simulink library "HEV_lib"  (Simulink 7.7)
settings: Solver=ode45  SolverMode=SingleTasking  StartTime=0.0  StopTime=10.0  RelTol=1e-3
undefined symbols (not defined in the file): DiscIntNeverNeededParam, Hydride, magnitude, Metal, Nickel, Ts
libraries: powerlib x72, driveline x12, simulink_extras x8, electricdrivelib x7, simulink x6, powerlib_extras x2, HEV_lib x1
(part 1 of 3)
Description:
  | Copyright 2008-2011 The MathWorks, Inc.
settings Model: Creator=MathWorks  LastModifiedBy=xd1824

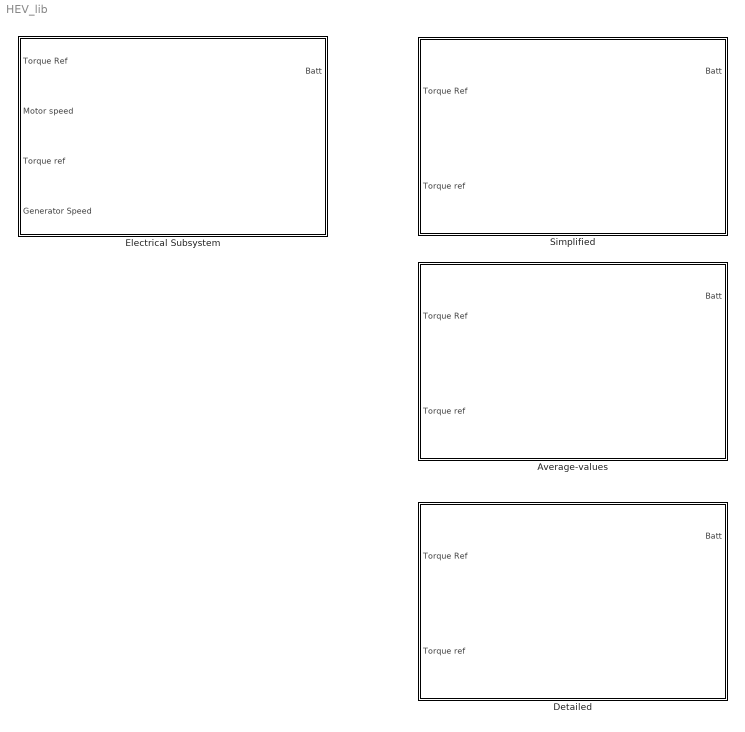
== system HEV_lib ==
  Average-values : Subsystem
      mask Display: image(imread('power_HEV_powertrain_electrical2.png'))
  Detailed : Subsystem
      mask Display: image(imread('power_HEV_powertrain_electrical2.png'))
  Electrical Subsystem : Subsystem  BlockChoice=Simplified
      settings: TemplateBlock=self  MemberBlocks=Average-values,Detailed,Simplified
      mask Display: image(imread('power_HEV_powertrain_electrical2.png'))
  Simplified : Subsystem
      mask Display: image(imread('power_HEV_powertrain_electrical2.png'))

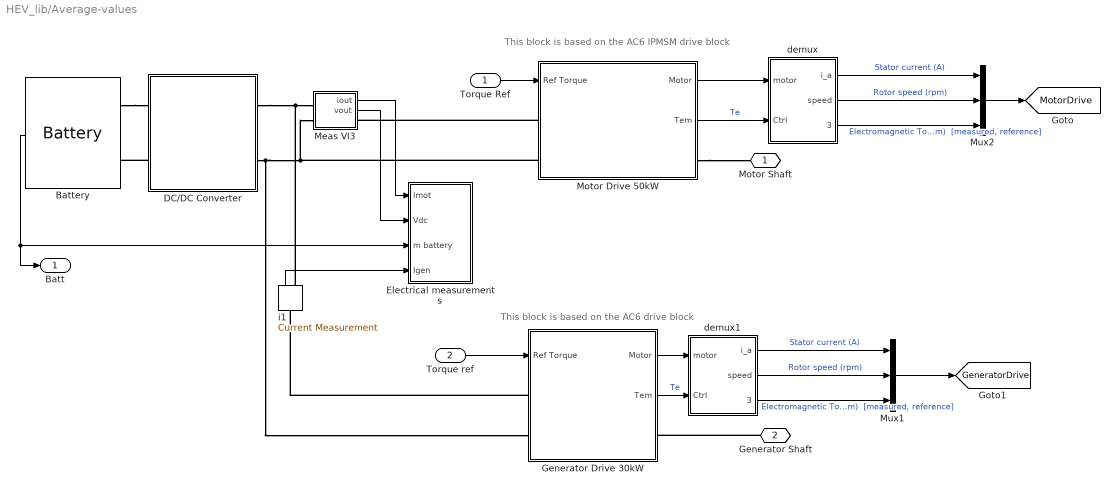
== system HEV_lib/Average-values ==
  note: This block is based on the
      | AC6 IPMSM drive block
  note: This block is based on the AC6
      | drive block
  Torque Ref : Inport
  Torque ref : Inport  Port=2
  Battery : electricdrivelib/Extra Sources/Battery  SystemSampleTime=-1  BatType=Nickel-Metal-Hydride  ShowDetailedParameters=off  NomV=200  NomQ=6.5  SOC=100  PresetModel=on  MaxQ=7  FullV=235.5932  Dis_rate=1.3  R=0.30769  Normal_OP=6.25  expZone="[216.9492           1.3]"  Dis_Char=off  current=[50 100]  Units=Time  Batt_Tr=30
  DC/DC Converter : Subsystem
      mask init:
      | [X1,X1m,X2,X2m,X3,X4,Y1,Y1m,Y2,Y2m,Y3,Y4,color1,color2]=spsdrivelogo;
      mask Display:
      | patch([X1 X1m],[Y1 Y1m],color1);
      | patch(X3,Y3,color2);
      | plot([X1 X1m X2 X2m X3 X4],[Y1 Y1m Y2 Y2m Y3 Y4]);
  Electrical measurements : Subsystem
  Generator Drive 30kW : Subsystem
      mask Display: image(imread('power_HEV_powertrain_syncgenerator.jpg'))
  Meas VI3 : Subsystem
  Motor Drive 50kW : Subsystem
      mask Display: image(imread('power_HEV_powertrain_syncmotor.jpg'))
  Mux1 : Mux  Inputs=3
  Mux2 : Mux  Inputs=3
  demux : Subsystem
  demux1 : Subsystem
  i1 : powerlib/Measurements/Current Measurement  SystemSampleTime=-1  PhasorSimulation=off  OutputType=Complex  PSBequivalent=0
  Motor Shaft : PMIOPort  Port=1  Side=Right
  Generator Shaft : PMIOPort  Port=2  Side=Right
  Batt : Outport
  tag scope: GeneratorDrive=global, MotorDrive=global
  wires:
  i1/1 -> Electrical measurements/4(Igen)
  Meas VI3/2(vout) -> Electrical measurements/2(Vdc)
  Meas VI3/1(iout) -> Electrical measurements/1(Imot)
  Torque ref/1 -> Generator Drive 30kW/1(Ref Torque)
  Battery/1 -> Electrical measurements/3(m battery), Batt/1
  demux1/2(speed) -> Mux1/2  "Rotor speed (rpm)"
  demux1/3(Torque) -> Mux1/3  "Electromagnetic Torque (Nm)  [measured, reference]"
  demux1/1(i_a) -> Mux1/1  "Stator current (A)"
  Generator Drive 30kW/1(Motor) -> demux1/1(motor)
  Torque Ref/1 -> Motor Drive 50kW/1(Ref Torque)
  Motor Drive 50kW/1(Motor) -> demux/1(motor)
  demux/2(speed) -> Mux2/2  "Rotor speed (rpm)"
  demux/3(Torque) -> Mux2/3  "Electromagnetic Torque (Nm)  [measured, reference]"
  demux/1(i_a) -> Mux2/1  "Stator current (A)"
  Mux2/1 -> [MotorDrive]
  Mux1/1 -> [GeneratorDrive]
  Motor Drive 50kW/2(Tem) -> demux/2(Ctrl)  "Te"
  Generator Drive 30kW/2(Tem) -> demux1/2(Ctrl)  "Te"
  connections:
  DC/DC Converter/LConn2 -- Battery/LConn2
  Battery/LConn1 -- DC/DC Converter/LConn1
  Generator Shaft/RConn1 -- Generator Drive 30kW/RConn1
  Motor Drive 50kW/LConn1 -- Meas VI3/RConn1
  DC/DC Converter/RConn1 -- Meas VI3/LConn1 -- i1/RConn1
  Generator Drive 30kW/LConn1 -- i1/LConn1
  DC/DC Converter/RConn2 -- Generator Drive 30kW/LConn2 -- Motor Drive 50kW/LConn2 -- Meas VI3/LConn2
  Motor Drive 50kW/RConn1 -- Motor Shaft/RConn1

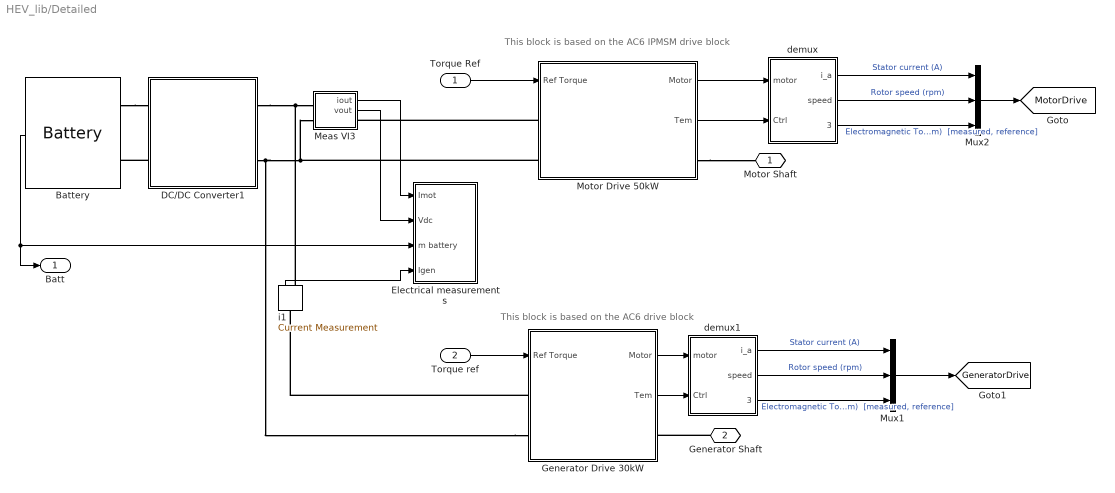
== system HEV_lib/Detailed ==
  note: This block is based on the AC6
      | drive block
  note: This block is based on the
      | AC6 IPMSM drive block
  Torque Ref : Inport
  Torque ref : Inport  Port=2
  Battery : electricdrivelib/Extra Sources/Battery  SystemSampleTime=-1  BatType=Nickel-Metal-Hydride  ShowDetailedParameters=off  NomV=200  NomQ=6.5  SOC=100  PresetModel=on  MaxQ=7  FullV=235.5932  Dis_rate=1.3  R=0.30769  Normal_OP=6.25  expZone="[216.9492           1.3]"  Dis_Char=off  current=[50 100]  Units=Time  Batt_Tr=30
  DC/DC Converter1 : Subsystem
      mask init:
      | [X1,X1m,X2,X2m,X3,X4,Y1,Y1m,Y2,Y2m,Y3,Y4,color1,color2]=spsdrivelogo;
      mask Display:
      | patch([X1 X1m],[Y1 Y1m],color1);
      | patch(X3,Y3,color2);
      | plot([X1 X1m X2 X2m X3 X4],[Y1 Y1m Y2 Y2m Y3 Y4]);
  Electrical measurements : Subsystem
  Generator Drive 30kW : Subsystem
      mask Display: image(imread('power_HEV_powertrain_syncgenerator.jpg'))
  Meas VI3 : Subsystem
  Motor Drive 50kW : Subsystem
      mask Display: image(imread('power_HEV_powertrain_syncmotor.jpg'))
  Mux1 : Mux  Inputs=3
  Mux2 : Mux  Inputs=3
  demux : Subsystem
  demux1 : Subsystem
  i1 : powerlib/Measurements/Current Measurement  SystemSampleTime=-1  PhasorSimulation=off  OutputType=Complex  PSBequivalent=0
  Motor Shaft : PMIOPort  Port=1  Side=Right
  Generator Shaft : PMIOPort  Port=2  Side=Right
  Batt : Outport
  tag scope: GeneratorDrive=global, MotorDrive=global
  wires:
  demux/1(i_a) -> Mux2/1  "Stator current (A)"
  demux/3(Torque) -> Mux2/3  "Electromagnetic Torque (Nm)  [measured, reference]"
  demux/2(speed) -> Mux2/2  "Rotor speed (rpm)"
  Motor Drive 50kW/2(Tem) -> demux/2(Ctrl)
  Motor Drive 50kW/1(Motor) -> demux/1(motor)
  Torque Ref/1 -> Motor Drive 50kW/1(Ref Torque)
  Generator Drive 30kW/2(Tem) -> demux1/2(Ctrl)
  Generator Drive 30kW/1(Motor) -> demux1/1(motor)
  demux1/1(i_a) -> Mux1/1  "Stator current (A)"
  demux1/3(Torque) -> Mux1/3  "Electromagnetic Torque (Nm)  [measured, reference]"
  demux1/2(speed) -> Mux1/2  "Rotor speed (rpm)"
  Battery/1 -> Batt/1, Electrical measurements/3(m battery)
  Torque ref/1 -> Generator Drive 30kW/1(Ref Torque)
  Meas VI3/1(iout) -> Electrical measurements/1(Imot)
  Meas VI3/2(vout) -> Electrical measurements/2(Vdc)
  i1/1 -> Electrical measurements/4(Igen)
  Mux2/1 -> [MotorDrive]
  Mux1/1 -> [GeneratorDrive]
  connections:
  Motor Drive 50kW/RConn1 -- Motor Shaft/RConn1
  Generator Drive 30kW/LConn2 -- Meas VI3/LConn2 -- Motor Drive 50kW/LConn2 -- DC/DC Converter1/RConn2
  Generator Drive 30kW/LConn1 -- i1/LConn1
  DC/DC Converter1/RConn1 -- i1/RConn1 -- Meas VI3/LConn1
  Motor Drive 50kW/LConn1 -- Meas VI3/RConn1
  Generator Shaft/RConn1 -- Generator Drive 30kW/RConn1
  Battery/LConn1 -- DC/DC Converter1/LConn1
  DC/DC Converter1/LConn2 -- Battery/LConn2

== system HEV_lib/Electrical Subsystem ==
  Torque Ref : Inport
  Motor speed : Inport  Port=2
  Torque ref : Inport  Port=3
  Generator Speed : Inport  Port=4
  Simplified : HEV_lib/Simplified  SystemSampleTime=-1
  Motor Shaft : PMIOPort  Port=1  Side=Right
  Generator Shaft : PMIOPort  Port=2  Side=Right
  Batt : Outport
  wires:
  Torque Ref/1 -> Simplified/1
  Motor speed/1 -> Simplified/2
  Torque ref/1 -> ?
  Generator Speed/1 -> ?
  Simplified/1 -> Batt/1
  connections:
  Simplified/RConn1 -- Motor Shaft/RConn1
  Simplified/RConn2 -- Generator Shaft/RConn1

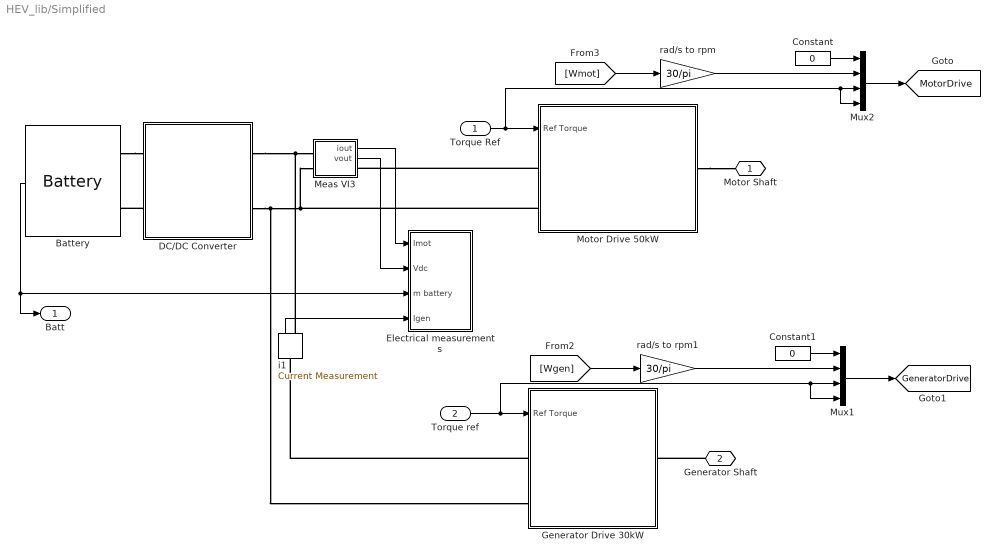
== system HEV_lib/Simplified ==
  Torque Ref : Inport
  Torque ref : Inport  Port=2
  Battery : electricdrivelib/Extra Sources/Battery  SystemSampleTime=-1  BatType=Nickel-Metal-Hydride  ShowDetailedParameters=off  NomV=200  NomQ=6.5  SOC=100  PresetModel=on  MaxQ=7  FullV=235.5932  Dis_rate=1.3  R=0.30769  Normal_OP=6.25  expZone="[216.9492           1.3]"  Dis_Char=off  current=[50 100]  Units=Time  Batt_Tr=30
  Constant : Constant  Value=0
  Constant1 : Constant  Value=0
  DC/DC Converter : Subsystem
      mask init:
      | [X1,X1m,X2,X2m,X3,X4,Y1,Y1m,Y2,Y2m,Y3,Y4,color1,color2]=spsdrivelogo;
      mask Display:
      | patch([X1 X1m],[Y1 Y1m],color1);
      | patch(X3,Y3,color2);
      | plot([X1 X1m X2 X2m X3 X4],[Y1 Y1m Y2 Y2m Y3 Y4]);
  Electrical measurements : Subsystem
  Generator Drive 30kW : Subsystem
      mask Display: image(imread('power_HEV_powertrain_syncgenerator.jpg'))
  Meas VI3 : Subsystem
  Motor Drive 50kW : Subsystem
      mask Display: image(imread('power_HEV_powertrain_syncmotor.jpg'))
  Mux1 : Mux
  Mux2 : Mux
  i1 : powerlib/Measurements/Current Measurement  SystemSampleTime=-1  PhasorSimulation=off  OutputType=Complex  PSBequivalent=0
  rad/s to rpm : Gain  Gain=30/pi
  rad/s to rpm1 : Gain  Gain=30/pi
  Motor Shaft : PMIOPort  Port=1  Side=Right
  Generator Shaft : PMIOPort  Port=2  Side=Right
  Batt : Outport
  tag scope: GeneratorDrive=global, MotorDrive=global
  wires:
  i1/1 -> Electrical measurements/4(Igen)
  Meas VI3/2(vout) -> Electrical measurements/2(Vdc)
  Meas VI3/1(iout) -> Electrical measurements/1(Imot)
  Torque ref/1 -> Generator Drive 30kW/1(Ref Torque), Mux1/3, Mux1/4
  Battery/1 -> Electrical measurements/3(m battery), Batt/1
  Torque Ref/1 -> Motor Drive 50kW/1(Ref Torque), Mux2/3, Mux2/4
  Mux2/1 -> [MotorDrive]
  rad/s to rpm/1 -> Mux2/2
  Constant/1 -> Mux2/1
  rad/s to rpm1/1 -> Mux1/2
  Constant1/1 -> Mux1/1
  Mux1/1 -> [GeneratorDrive]
  [Wmot] -> rad/s to rpm/1
  [Wgen] -> rad/s to rpm1/1
  connections:
  DC/DC Converter/LConn2 -- Battery/LConn2
  Battery/LConn1 -- DC/DC Converter/LConn1
  Generator Shaft/RConn1 -- Generator Drive 30kW/RConn1
  DC/DC Converter/RConn1 -- Meas VI3/LConn1 -- i1/RConn1
  DC/DC Converter/RConn2 -- Meas VI3/LConn2 -- Motor Drive 50kW/LConn2 -- Generator Drive 30kW/LConn2
  Motor Drive 50kW/RConn1 -- Motor Shaft/RConn1
  Motor Drive 50kW/LConn1 -- Meas VI3/RConn1
  Generator Drive 30kW/LConn1 -- i1/LConn1

== system HEV_lib/Average-values/DC/DC Converter ==
  Average-values Boost Converter : Subsystem  mask(SPSdrives Converter){SnubberResistance=10e3, SnubberCapacitance=inf, Ron=1e-3, ForwardVoltages=[1.3,1.3], IGBTParameters=[0,0], converterType=Inverter}
      mask prompts: SnubberResistance "Snubber resistance Rs (Ohms):"; SnubberCapacitance "Snubber capacitance Cs (F):"; Ron "Ron (Ohms):"; ForwardVoltages "Forward voltages [Device Vf(V), Diode Vd (V)]"; IGBTParameters "[Tf(s), Tt(s)]:"; converterType "Converter type:"
      mask help: This model implements an average-value buck converter."Duty Cycle" contains the duty cycle of the internal IGBT device.
      mask StyleString: edit,edit,edit,edit,edit,popup(Rectifier|Inverter)
      mask Display: plot(0,0,100,100,[39 39 23.8],[71 28 28],[44 56 49.6 56 52.8 56 61 61],[39.2 33.6 32.8 33.6 40.8 33.6 30 12.4],[44 44 44 61 61],[28 71 60 66.4 90],[75 67 83 75 67 83 75 75],[54 42 42 54 54 54 54 66],[61 75 75],[24 24 42],[75 75 61],[66,76,76])
  CBus : powerlib/Elements/Series RLC Branch  PhysicalDomain=powersysdomain  SubClassName=unknown  LeftPortType=p1  RightPortType=p1  LConnTagsString=__new0  RConnTagsString=__new0  BranchType=RC  Resistance=0.1  Inductance=1e-3  SetiL0=off  InitialCurrent=0  Capacitance=1130e-6  Setx0=on  InitialVoltage=500  Measurements=None
  CBus1 : powerlib/Elements/Series RLC Branch  PhysicalDomain=powersysdomain  SubClassName=unknown  LeftPortType=p1  RightPortType=p1  LConnTagsString=__new0  RConnTagsString=__new0  BranchType=C  Resistance=0.2  Inductance=1e-3  SetiL0=off  InitialCurrent=0  Capacitance=282e-6  Setx0=on  InitialVoltage=150  Measurements=None
  Current controller DISCRETE3 : Subsystem  mask(PI controller){Kp=0.001, Ki=1, Ts=Ts}
      mask prompts: Kp "Proportional gain (Kp)"; Ki "Integral gain (Ki)"; Ts "Sample time (s) :"
      mask help: Proportional-Integral Speed Controller
      mask Display: plot(0,0,100,100,[35,35,65],[70,30,30],[35,65],[45,60])
  Duty Cycles : Subsystem
  L : powerlib/Elements/Series RLC Branch  PhysicalDomain=powersysdomain  SubClassName=unknown  LeftPortType=p1  RightPortType=p1  LConnTagsString=__new0  RConnTagsString=__new0  BranchType=L  Resistance=0.3  Inductance=373e-6  SetiL0=off  InitialCurrent=100  Capacitance=100e-6  Setx0=off  InitialVoltage=0  Measurements=None
  Mux1 : Mux  Inputs=2
  Ubus Ref : Constant  Value=500
  V1 : powerlib/Measurements/Voltage Measurement  SystemSampleTime=-1  PhasorSimulation=off  OutputType=Complex  PSBequivalent=0
  +Vdc Bus : PMIOPort  Tag=PMCPort  Port=1  Side=Right
  -Vdc Bus : PMIOPort  Tag=PMCPort  Port=2  Side=Right
  + battery : PMIOPort  Tag=PMCPort  Port=3  Side=Left
  - battery : PMIOPort  Tag=PMCPort  Port=4  Side=Left
  tag scope: V_DCDC=global
  wires:
  V1/1 -> Mux1/2, Current controller DISCRETE3/2(UBus)
  Ubus Ref/1 -> Mux1/1, Current controller DISCRETE3/1(Uref)
  Current controller DISCRETE3/1(Ec) -> Duty Cycles/1(Ec)
  Duty Cycles/1(dc) -> Average-values Boost Converter/1(Duty Cycle)
  Mux1/1 -> [V_DCDC]
  connections:
  L/RConn1 -- + battery/RConn1 -- CBus1/LConn1
  V1/LConn2 -- CBus/RConn1 -- -Vdc Bus/RConn1 -- - battery/RConn1 -- CBus1/RConn1 -- Average-values Boost Converter/LConn2
  V1/LConn1 -- CBus/LConn1 -- Average-values Boost Converter/LConn1 -- +Vdc Bus/RConn1
  L/LConn1 -- Average-values Boost Converter/RConn1

== system HEV_lib/Average-values/Electrical measurements ==
  Imot : Inport
  Vdc : Inport  Port=2
  m battery : Inport  Port=3
  Igen : Inport  Port=4
  Bus Selector : BusSelector  OutputSignals=Voltage (V),Current (A),SOC (%)
  Mux : Mux  Inputs=2
  Mux1 : Mux  Inputs=3
  Mux2 : Mux  Inputs=3
  Mux3 : Mux
  Product1 : Product  RndMeth=Zero
  Product2 : Product  RndMeth=Zero
  Product3 : Product  RndMeth=Zero
  tag scope: Electricals=global, Power=global
  wires:
  Product2/1 -> Mux1/1  "Motor Power (W)"
  Product1/1 -> Mux1/2  "Generator power (W)"
  Product3/1 -> Mux1/3  "Battery power (W)"
  Imot/1 -> Product2/1, Mux2/1
  Mux1/1 -> [Power]
  m battery/1 -> Bus Selector/1
  Bus Selector/1 -> Mux/2, Product3/1  "<Voltage (V)>"
  Bus Selector/2 -> Product3/2, Mux2/2  "<Current (A)>"
  [V_DCDC] -> Mux3/1  "DC/DC converter Voltage (Reference, Measured)"
  Mux/1 -> Mux3/2  "Voltage (DC bus, Battery)"
  Mux2/1 -> Mux3/3  "Current (Motor, Battery, Generator)"
  Igen/1 -> Product1/1, Mux2/3
  Bus Selector/3 -> Mux3/4  "<SOC (%)>"
  Vdc/1 -> Product2/2, Product1/2, Mux/1
  Mux3/1 -> [Electricals]

== system HEV_lib/Average-values/Generator Drive 30kW ==
  Ref Torque : Inport
  Bus Selector : BusSelector  OutputSignals=Rotor angle thetam (rad),Electromagnetic torque Te (N*m)
  Measures : electricdrivelib/AC drives/PM Synchronous Motor Drive/Measures  SystemSampleTime=-1
  Mux : Subsystem
  PMSM1 : powerlib/Machines/Permanent Magnet Synchronous Machine  SystemSampleTime=-1  NbPhases=3  FluxDistribution=Sinusoidal  RotorType=Salient-pole  MechanicalLoad=Speed w  PresetModel=No  ShowDetailedParameters=on  Resistance=0.05  Inductance=0  dqInductances=[0.000635 0.000635]  La=0.000835  MachineConstant=Flux linkage established by magnets (V.s)  Flux=0.192  VoltageCst=34.8249  TorqueCst=0.288  Flat=0  Mechanical=[0.011 0.001889/4 4/4]  PolePairs=1  InitialConditions=[0,0, 0,0,0]  InitialConditions5ph=[0 0 0 0 0 0]  TsPowergui=0  TsBlock=-1
      settings: AttributesFormatString=\n
  SIm/SDL : driveline/Sensors & Actuators/Torque Actuator  SystemSampleTime=-1
  Speed Sensor : driveline/Sensors & Actuators/Motion Sensor  SystemSampleTime=-1  Angle=off  x0=0  Velocity=on  Acceleration=off
  Three-phase Inverter : Subsystem  mask(SPSdrives Converter){Arms=3, SnubberResistance=5000, SnubberCapacitance=inf, Device=IGBT / Diodes, Ron=1e-3, Lon=0, ForwardVoltages=[0.8,0.8], ForwardVoltage=0, GTOparameters=[0,0], IGBTparameters=[1e-6,2e-6], Measurements=All voltages and currents, SourceFrequency=60, dqInductances=[0.000635,0.000635], Flux=0.192, Resistance=0.05, p=4/4, converterType=Inverter}
      mask prompts: Arms "Number of bridge arms:"; SnubberResistance "Snubber resistance Rs (Ohms)"; SnubberCapacitance "Snubber capacitance Cs (F)"; Device "Power Electronic device"; Ron "Ron (Ohms)"; Lon "Lon (H)"; ForwardVoltages "Forward voltages  [ Device Vf(V) , Diode Vfd(V)]"; ForwardVoltage "Forward voltage Vf (V)"; GTOparameters "[  Tf (s) , Tt (s)  ]"; IGBTparameters "[  Tf (s) , Tt (s)  ]"; SourceFrequency "Source Frequency (Hz)"; dqInductances "PMSM-Inductances [ Ld(H) Lq(H) ]:"; Flux "PMSM-Flux induced by magnets (Wb):"; Resistance "PMSM-Stator resistance Rs (ohm):"; p "PMSM-Pairs of poles p:"; converterType "Converter type:"
      mask init:
      | Ld=dqInductances(1);
      | Lq=dqInductances(2);
      | Fcs=6*SourceFrequency/10;
      settings: OpenFcn=power_openblockproxy();
      mask Help: web(psbhelp);
      mask StyleString: popup(1|2|3),edit,edit,popup(Diodes|Thyristors|GTO / Diodes|MOSFET / Diodes|IGBT / Diodes|Ideal Switches),edit,edit,edit,edit,edit,edit,popup(None|Device voltages|Device currents|UAB UBC UCA UDC voltages|All voltages and currents),edit,edit,edit,edit,edit,popup(Rectifier|Inverter)
      mask Display: plot(0,0,100,100,[39 39 23.8],[71 28 28],[44 56 49.6 56 52.8 56 61 61],[39.2 33.6 32.8 33.6 40.8 33.6 30 12.4],[44 44 44 61 61],[28 71 60 66.4 90],[75 67 83 75 67 83 75 75],[54 42 42 54 54 54 54 66],[61 75 75],[24 24 42],[75 75 61],[66,76,76])
  VECT : Subsystem  mask(VECT){nb_p=4/4, lambda=0.192, freq_max=20e3, Ts_vect=60e-6, h=2}
      mask prompts: nb_p "Motor pairs of poles"; lambda "Flux induced by magnets (Wb)"; freq_max "Maximum switching frequency (Hz)"; Ts_vect "Sampling time (s)"; h "Current hysteresis bandwidth (A)"
      mask help: This block implements a vector controller.
      mask init:
      | [X1,X1m,X2,X2m,X3,X4,Y1,Y1m,Y2,Y2m,Y3,Y4,color1,color2]=spsdrivelogo;
      mask Display:
      | patch([X1 X1m],[Y1 Y1m],color1);
      | patch(X3,Y3,color2);
      | plot([X1 X1m X2 X2m X3 X4],[Y1 Y1m Y2 Y2m Y3 Y4]);
  + : PMIOPort  Port=1  Side=Left
  - : PMIOPort  Port=2  Side=Left
  Generator Shaft : PMIOPort  Port=3  Side=Right
  Motor : Outport
  Tem : Outport  Port=2
  wires:
  Speed Sensor/1 -> PMSM1/1
  Measures/1 -> VECT/3(I_abc)
  VECT/1(sig*) -> Mux/1(sig*)
  Mux/1(Ctrl) -> Three-phase Inverter/1(ctrl)
  Ref Torque/1 -> VECT/1(Torque*)
  PMSM1/1 -> Motor/1, Bus Selector/1, Mux/2(m)
  Bus Selector/1 -> VECT/2(teta)  "<Rotor angle thetam (rad)>"
  Bus Selector/2 -> Tem/1, SIm/SDL/1  "<Electromagnetic torque Te (N*m)>"
  connections:
  -/RConn1 -- Three-phase Inverter/RConn2
  +/RConn1 -- Three-phase Inverter/RConn1
  Measures/RConn1 -- PMSM1/LConn1
  Measures/RConn2 -- PMSM1/LConn2
  Measures/RConn3 -- PMSM1/LConn3
  Three-phase Inverter/LConn1 -- Measures/LConn1
  Measures/LConn2 -- Three-phase Inverter/LConn2
  Three-phase Inverter/LConn3 -- Measures/LConn3
  Generator Shaft/RConn1 -- SIm/SDL/RConn1 -- Speed Sensor/LConn1

== system HEV_lib/Average-values/Meas VI3 ==
  V1 : powerlib/Measurements/Voltage Measurement  SystemSampleTime=-1  PhasorSimulation=off  OutputType=Complex  PSBequivalent=0
  i1 : powerlib/Measurements/Current Measurement  SystemSampleTime=-1  PhasorSimulation=off  OutputType=Complex  PSBequivalent=0
  iref : PMIOPort  Port=1  Side=Right
  + : PMIOPort  Tag=PMCPort  Port=2  Side=Left
  vref : PMIOPort  Port=3  Side=Left
  iout : Outport
  vout : Outport  Port=2
  wires:
  V1/1 -> vout/1
  i1/1 -> iout/1
  connections:
  vref/RConn1 -- V1/LConn2
  iref/RConn1 -- i1/RConn1
  i1/LConn1 -- +/RConn1 -- V1/LConn1

== system HEV_lib/Average-values/Motor Drive 50kW ==
  Ref Torque : Inport
  500 Vdc 50kW PMSM : powerlib/Machines/Permanent Magnet Synchronous Machine  SystemSampleTime=-1  NbPhases=3  FluxDistribution=Sinusoidal  RotorType=Salient-pole  MechanicalLoad=Speed w  PresetModel=No  ShowDetailedParameters=on  Resistance=0.0065  Inductance=0  dqInductances="[0.001597972349731   0.002057052250467]"  La=0.000835  MachineConstant=Flux linkage established by magnets (V.s)  Flux=0.175666143629361  VoltageCst=127.4493  TorqueCst=1.054  Flat=0  Mechanical=[0.089 0.005 4]  PolePairs=4  InitialConditions=[0,0,0,0]  InitialConditions5ph=[0 0 0 0 0 0]  TsPowergui=0  TsBlock=-1
      settings: AttributesFormatString=\n
  Bus Selector : BusSelector  OutputSignals=Rotor speed wm (rad/s),Rotor angle thetam (rad),Electromagnetic torque Te (N*m)
  Measures : electricdrivelib/AC drives/PM Synchronous Motor Drive/Measures  SystemSampleTime=-1
  Mux : Subsystem
  SIm/SDL1 : driveline/Sensors & Actuators/Torque Actuator  SystemSampleTime=-1
  Speed Sensor : driveline/Sensors & Actuators/Motion Sensor  SystemSampleTime=-1  Angle=off  x0=0  Velocity=on  Acceleration=off
  Three-phase Inverter : Subsystem  mask(SPSdrives Converter){Arms=3, SnubberResistance=5000, SnubberCapacitance=inf, Device=IGBT / Diodes, Ron=1e-3, Lon=0, ForwardVoltages=[0.8,0.8], ForwardVoltage=0, GTOparameters=[0,0], IGBTparameters=[1e-6,2e-6], Measurements=All voltages and currents, SourceFrequency=60, dqInductances=[0.001597972349731   0.002057052250467], Flux=0.175666143629361, Resistance=0.0065, p=4, converterType=Inverter}
      mask prompts: Arms "Number of bridge arms:"; SnubberResistance "Snubber resistance Rs (Ohms)"; SnubberCapacitance "Snubber capacitance Cs (F)"; Device "Power Electronic device"; Ron "Ron (Ohms)"; Lon "Lon (H)"; ForwardVoltages "Forward voltages  [ Device Vf(V) , Diode Vfd(V)]"; ForwardVoltage "Forward voltage Vf (V)"; GTOparameters "[  Tf (s) , Tt (s)  ]"; IGBTparameters "[  Tf (s) , Tt (s)  ]"; SourceFrequency "Source Frequency (Hz)"; dqInductances "PMSM-Inductances [ Ld(H) Lq(H) ]:"; Flux "PMSM-Flux induced by magnets (Wb):"; Resistance "PMSM-Stator resistance Rs (ohm):"; p "PMSM-Pairs of poles p:"; converterType "Converter type:"
      mask init:
      | Ld=dqInductances(1);
      | Lq=dqInductances(2);
      | Fcs=6*SourceFrequency/10;
      settings: OpenFcn=power_openblockproxy();
      mask Help: web(psbhelp);
      mask StyleString: popup(1|2|3),edit,edit,popup(Diodes|Thyristors|GTO / Diodes|MOSFET / Diodes|IGBT / Diodes|Ideal Switches),edit,edit,edit,edit,edit,edit,popup(None|Device voltages|Device currents|UAB UBC UCA UDC voltages|All voltages and currents),edit,edit,edit,edit,edit,popup(Rectifier|Inverter)
      mask Display: plot(0,0,100,100,[39 39 23.8],[71 28 28],[44 56 49.6 56 52.8 56 61 61],[39.2 33.6 32.8 33.6 40.8 33.6 30 12.4],[44 44 44 61 61],[28 71 60 66.4 90],[75 67 83 75 67 83 75 75],[54 42 42 54 54 54 54 66],[61 75 75],[24 24 42],[75 75 61],[66,76,76])
  Torque limitation : Subsystem
      mask Display: plot([0;1800;2000;2500;3000;3500], [1;1;0.90*1;0.72*1;0.6*1;0.51*1])
  VECT controller : Subsystem  mask(VECT){nb_p=4, dqInductances=[0.001597972349731   0.002057052250467], lambda=0.175666143629361, Ts_vect=60e-6}
      mask prompts: nb_p "Motor pairs of poles"; dqInductances "Inductances [ Ld(H) Lq(H) ]:"; lambda "Flux induced by magnets (Wb)"; Ts_vect "Sampling time (s)"
      mask help: This block implements a vector controller.
      mask init:
      | [X1,X1m,X2,X2m,X3,X4,Y1,Y1m,Y2,Y2m,Y3,Y4,color1,color2]=spsdrivelogo;
      | ib = lambda/(dqInductances(2)-dqInductances(1));
      | Teb = 3/2*nb_p*lambda*ib;
      | Ld = dqInductances(1);
      | Lq = dqInductances(2);
      | lam = lambda;
      | p=nb_p;
      | ib = lam/(Lq-Ld);
      | iqn = 0:0.01:3;
      | ten = iqn/2.*(sqrt(4*iqn.*iqn+1)+1);
      mask Display:
      | patch([X1 X1m],[Y1 Y1m],color1);
      | patch(X3,Y3,color2);
      | plot([X1 X1m X2 X2m X3 X4],[Y1 Y1m Y2 Y2m Y3 Y4]);
  +Vdc Bus : PMIOPort  Port=1  Side=Left
  -Vdc Bus : PMIOPort  Port=2  Side=Left
  Motor Shaft : PMIOPort  Port=3  Side=Right
  Motor : Outport
  Tem : Outport  Port=2
  wires:
  Mux/1(Ctrl) -> Three-phase Inverter/1(ctrl)
  VECT controller/1(sig*) -> Mux/1(sig*)
  Speed Sensor/1 -> 500 Vdc 50kW PMSM/1
  500 Vdc 50kW PMSM/1 -> Bus Selector/1, Mux/2(m), Motor/1
  Bus Selector/3 -> Tem/1, SIm/SDL1/1  "<Electromagnetic torque Te (N*m)>"
  Bus Selector/1 -> VECT controller/2(w), Torque limitation/1(N rad/s)  "<Rotor speed wm (rad/s)>"
  Measures/1 -> VECT controller/4(I_abc)
  Bus Selector/2 -> VECT controller/3(teta)  "<Rotor angle thetam (rad)>"
  Torque limitation/1(torque) -> VECT controller/1(Torque*)
  Ref Torque/1 -> Torque limitation/2(Torque)
  connections:
  Three-phase Inverter/LConn3 -- Measures/LConn3
  Measures/LConn2 -- Three-phase Inverter/LConn2
  Three-phase Inverter/LConn1 -- Measures/LConn1
  Measures/RConn3 -- 500 Vdc 50kW PMSM/LConn3
  Measures/RConn2 -- 500 Vdc 50kW PMSM/LConn2
  Measures/RConn1 -- 500 Vdc 50kW PMSM/LConn1
  +Vdc Bus/RConn1 -- Three-phase Inverter/RConn1
  -Vdc Bus/RConn1 -- Three-phase Inverter/RConn2
  SIm/SDL1/RConn1 -- Motor Shaft/RConn1 -- Speed Sensor/LConn1

== system HEV_lib/Average-values/demux ==
  motor : Inport
  Ctrl : Inport  Port=2
  "+ -> -1" : Gain  Gain=30/pi
  Bus Selector : BusSelector  OutputSignals=Stator current is_a (A),Rotor speed wm (rad/s),Electromagnetic torque Te (N*m)
  Mux1 : Mux  Inputs=2
  i_a : Outport
  speed : Outport  Port=2
  Torque : Outport  Port=3
  wires:
  "+ -> -1"/1 -> speed/1
  motor/1 -> Bus Selector/1
  Ctrl/1 -> Mux1/2
  Bus Selector/2 -> "+ -> -1"/1  "<Rotor speed wm (rad/s)>"
  Bus Selector/3 -> Mux1/1  "<Electromagnetic torque Te (N*m)>"
  Mux1/1 -> Torque/1
  Bus Selector/1 -> i_a/1  "<Stator current is_a (A)>"

== system HEV_lib/Average-values/demux1 ==
  motor : Inport
  Ctrl : Inport  Port=2
  "+ -> -1" : Gain  Gain=30/pi
  Bus Selector : BusSelector  OutputSignals=Stator current is_a (A),Rotor speed wm (rad/s),Electromagnetic torque Te (N*m)
  Mux1 : Mux  Inputs=2
  i_a : Outport
  speed : Outport  Port=2
  Torque : Outport  Port=3
  wires:
  Mux1/1 -> Torque/1
  Bus Selector/3 -> Mux1/1  "<Electromagnetic torque Te (N*m)>"
  Bus Selector/2 -> "+ -> -1"/1  "<Rotor speed wm (rad/s)>"
  Ctrl/1 -> Mux1/2
  Bus Selector/1 -> i_a/1  "<Stator current is_a (A)>"
  motor/1 -> Bus Selector/1
  "+ -> -1"/1 -> speed/1

== system HEV_lib/Detailed/DC/DC Converter1 ==
  CBus : powerlib/Elements/Series RLC Branch  PhysicalDomain=powersysdomain  SubClassName=unknown  LeftPortType=p1  RightPortType=p1  LConnTagsString=__new0  RConnTagsString=__new0  BranchType=RC  Resistance=0.1  Inductance=1e-3  SetiL0=off  InitialCurrent=0  Capacitance=1130e-6  Setx0=on  InitialVoltage=500  Measurements=None
  CBus1 : powerlib/Elements/Series RLC Branch  PhysicalDomain=powersysdomain  SubClassName=unknown  LeftPortType=p1  RightPortType=p1  LConnTagsString=__new0  RConnTagsString=__new0  BranchType=C  Resistance=0.2  Inductance=1e-3  SetiL0=off  InitialCurrent=0  Capacitance=282e-6  Setx0=on  InitialVoltage=150  Measurements=None
  Current controller DISCRETE3 : Subsystem  mask(PI controller){Kp=0.001, Ki=1, Ts=Ts}
      mask prompts: Kp "Proportional gain (Kp)"; Ki "Integral gain (Ki)"; Ts "Sample time (s) :"
      mask help: Proportional-Integral Speed Controller
      mask Display: plot(0,0,100,100,[35,35,65],[70,30,30],[35,65],[45,60])
  Detailed Boost converter : powerlib/Power Electronics/Universal Bridge  SystemSampleTime=-1  Arms=1  SnubberResistance=5000  SnubberCapacitance=inf  Device=IGBT / Diodes  Ron=1e-3  Lon=0  ForwardVoltages=[0,0]  ForwardVoltage=0  GTOparameters=[ 10e-6 , 20e-6 ]  IGBTparameters=[0,0]  Measurements=None  Measurements_2=None  converterType=Rectifier
  L : powerlib/Elements/Series RLC Branch  PhysicalDomain=powersysdomain  SubClassName=unknown  LeftPortType=p1  RightPortType=p1  LConnTagsString=__new0  RConnTagsString=__new0  BranchType=L  Resistance=0.3  Inductance=373e-6  SetiL0=off  InitialCurrent=100  Capacitance=100e-6  Setx0=off  InitialVoltage=0  Measurements=None
  Mux1 : Mux  Inputs=2
  PWM : Subsystem
  Ubus Ref : Constant  Value=500
  V1 : powerlib/Measurements/Voltage Measurement  SystemSampleTime=-1  PhasorSimulation=off  OutputType=Complex  PSBequivalent=0
  +Vdc Bus : PMIOPort  Tag=PMCPort  Port=1  Side=Right
  -Vdc Bus : PMIOPort  Tag=PMCPort  Port=2  Side=Right
  + battery : PMIOPort  Tag=PMCPort  Port=3  Side=Left
  - battery : PMIOPort  Tag=PMCPort  Port=4  Side=Left
  tag scope: V_DCDC=global
  wires:
  Mux1/1 -> [V_DCDC]
  PWM/1(Pulses) -> Detailed Boost converter/1
  Current controller DISCRETE3/1(Ec) -> PWM/1(Ref.)
  Ubus Ref/1 -> Current controller DISCRETE3/1(Uref), Mux1/1
  V1/1 -> Current controller DISCRETE3/2(UBus), Mux1/2
  connections:
  L/LConn1 -- Detailed Boost converter/LConn1
  Detailed Boost converter/RConn1 -- CBus/LConn1 -- V1/LConn1 -- +Vdc Bus/RConn1
  + battery/RConn1 -- L/RConn1 -- CBus1/LConn1
  Detailed Boost converter/RConn2 -- -Vdc Bus/RConn1 -- CBus/RConn1 -- V1/LConn2 -- - battery/RConn1 -- CBus1/RConn1

== system HEV_lib/Detailed/Electrical measurements ==
  Imot : Inport
  Vdc : Inport  Port=2
  m battery : Inport  Port=3
  Igen : Inport  Port=4
  Bus Selector : BusSelector  OutputSignals=Voltage (V),Current (A),SOC (%)
  Mux : Mux  Inputs=2
  Mux1 : Mux  Inputs=3
  Mux2 : Mux  Inputs=3
  Mux3 : Mux
  Product1 : Product  RndMeth=Zero
  Product2 : Product  RndMeth=Zero
  Product3 : Product  RndMeth=Zero
  Transfer Fcn : TransferFcn  Denominator=[.001 1]
  Transfer Fcn1 : TransferFcn  Denominator=[.001 1]
  Transfer Fcn2 : TransferFcn  Denominator=[.001 1]
  tag scope: Electricals=global, Power=global
  wires:
  Product2/1 -> Mux1/1  "Motor Power (W)"
  Product1/1 -> Mux1/2  "Generator power (W)"
  Product3/1 -> Mux1/3  "Battery power (W)"
  Imot/1 -> Transfer Fcn/1
  Mux1/1 -> [Power]
  m battery/1 -> Bus Selector/1
  Bus Selector/1 -> Mux/2, Product3/1  "<Voltage (V)>"
  Bus Selector/2 -> Transfer Fcn2/1  "<Current (A)>"
  [V_DCDC] -> Mux3/1  "DC/DC converter Voltage (Reference, Measured)"
  Mux/1 -> Mux3/2  "Voltage (DC bus, Battery)"
  Mux2/1 -> Mux3/3  "Current (Motor, Battery, Generator)"
  Igen/1 -> Transfer Fcn1/1
  Bus Selector/3 -> Mux3/4  "<SOC (%)>"
  Vdc/1 -> Product2/2, Product1/2, Mux/1
  Mux3/1 -> [Electricals]
  Transfer Fcn/1 -> Product2/1, Mux2/1
  Transfer Fcn1/1 -> Product1/1, Mux2/3
  Transfer Fcn2/1 -> Product3/2, Mux2/2

== system HEV_lib/Detailed/Generator Drive 30kW ==
  Ref Torque : Inport
  Bus Selector : BusSelector  OutputSignals=Rotor angle thetam (rad),Electromagnetic torque Te (N*m)
  Measures : electricdrivelib/AC drives/PM Synchronous Motor Drive/Measures  SystemSampleTime=-1
  Mux : Subsystem
  PMSM1 : powerlib/Machines/Permanent Magnet Synchronous Machine  SystemSampleTime=-1  NbPhases=3  FluxDistribution=Sinusoidal  RotorType=Salient-pole  MechanicalLoad=Speed w  PresetModel=No  ShowDetailedParameters=on  Resistance=0.05  Inductance=0  dqInductances=[0.000635 0.000635]  La=0.000835  MachineConstant=Flux linkage established by magnets (V.s)  Flux=0.192  VoltageCst=34.8249  TorqueCst=0.288  Flat=0  Mechanical=[0.011 0.001889/4 4/4]  PolePairs=1  InitialConditions=[0,0, 0,0,0]  InitialConditions5ph=[0 0 0 0 0 0]  TsPowergui=0  TsBlock=-1
      settings: AttributesFormatString=\n
  SIm/SDL : driveline/Sensors & Actuators/Torque Actuator  SystemSampleTime=-1
  Speed Sensor : driveline/Sensors & Actuators/Motion Sensor  SystemSampleTime=-1  Angle=off  x0=0  Velocity=on  Acceleration=off
  Three-phase Inverter : powerlib/Power Electronics/Universal Bridge  SystemSampleTime=-1  Arms=3  SnubberResistance=5000  SnubberCapacitance=inf  Device=IGBT / Diodes  Ron=1e-3  Lon=0  ForwardVoltages="[  0  0  ]"  ForwardVoltage=0  GTOparameters=[ 10e-6 , 20e-6 ]  IGBTparameters=[ 1e-6 , 2e-6 ]*0  Measurements=None  Measurements_2=None  converterType=Rectifier
  VECT : Subsystem  mask(VECT){nb_p=1, lambda=0.192, freq_max=20e3, Ts_vect=20e-6, h=0.1}
      mask prompts: nb_p "Motor pairs of poles"; lambda "Flux induced by magnets (Wb)"; freq_max "Maximum switching frequency (Hz)"; Ts_vect "Sampling time (s)"; h "Current hysteresis bandwidth (A)"
      mask help: This block implements a vector controller.
      mask init:
      | [X1,X1m,X2,X2m,X3,X4,Y1,Y1m,Y2,Y2m,Y3,Y4,color1,color2]=spsdrivelogo;
      mask Display:
      | patch([X1 X1m],[Y1 Y1m],color1);
      | patch(X3,Y3,color2);
      | plot([X1 X1m X2 X2m X3 X4],[Y1 Y1m Y2 Y2m Y3 Y4]);
  + : PMIOPort  Port=1  Side=Left
  - : PMIOPort  Port=2  Side=Left
  Generator Shaft : PMIOPort  Port=3  Side=Right
  Motor : Outport
  Tem : Outport  Port=2
  wires:
  Ref Torque/1 -> VECT/1(Torque*)
  Bus Selector/1 -> VECT/2(teta)  "<Rotor angle thetam (rad)>"
  Mux/1(g) -> Three-phase Inverter/1
  VECT/1(gates) -> Mux/1(gates)
  Measures/1 -> VECT/3(I_abc)
  Bus Selector/2 -> SIm/SDL/1, Tem/1  "<Electromagnetic torque Te (N*m)>"
  Speed Sensor/1 -> PMSM1/1
  PMSM1/1 -> Bus Selector/1, Mux/2(m), Motor/1
  connections:
  Generator Shaft/RConn1 -- SIm/SDL/RConn1 -- Speed Sensor/LConn1
  Three-phase Inverter/LConn3 -- Measures/LConn3
  Measures/LConn2 -- Three-phase Inverter/LConn2
  Three-phase Inverter/LConn1 -- Measures/LConn1
  Measures/RConn3 -- PMSM1/LConn3
  Measures/RConn2 -- PMSM1/LConn2
  Measures/RConn1 -- PMSM1/LConn1
  +/RConn1 -- Three-phase Inverter/RConn1
  -/RConn1 -- Three-phase Inverter/RConn2

== system HEV_lib/Detailed/Meas VI3 ==
  V1 : powerlib/Measurements/Voltage Measurement  SystemSampleTime=-1  PhasorSimulation=off  OutputType=Complex  PSBequivalent=0
  i1 : powerlib/Measurements/Current Measurement  SystemSampleTime=-1  PhasorSimulation=off  OutputType=Complex  PSBequivalent=0
  iref : PMIOPort  Port=1  Side=Right
  + : PMIOPort  Tag=PMCPort  Port=2  Side=Left
  vref : PMIOPort  Port=3  Side=Left
  iout : Outport
  vout : Outport  Port=2
  wires:
  i1/1 -> iout/1
  V1/1 -> vout/1
  connections:
  V1/LConn1 -- +/RConn1 -- i1/LConn1
  iref/RConn1 -- i1/RConn1
  vref/RConn1 -- V1/LConn2

== system HEV_lib/Detailed/Motor Drive 50kW ==
  Ref Torque : Inport
  500 Vdc 50kW PMSM : powerlib/Machines/Permanent Magnet Synchronous Machine  SystemSampleTime=-1  NbPhases=3  FluxDistribution=Sinusoidal  RotorType=Salient-pole  MechanicalLoad=Speed w  PresetModel=No  ShowDetailedParameters=on  Resistance=0.0065  Inductance=0  dqInductances="[0.001597972349731   0.002057052250467]"  La=0.000835  MachineConstant=Flux linkage established by magnets (V.s)  Flux=0.175666143629361  VoltageCst=127.4493  TorqueCst=1.054  Flat=0  Mechanical=[0.089 0.005 4]  PolePairs=4  InitialConditions=[0,0,0,0]  InitialConditions5ph=[0 0 0 0 0 0]  TsPowergui=0  TsBlock=-1
      settings: AttributesFormatString=\n
  Bus Selector : BusSelector  OutputSignals=Rotor speed wm (rad/s),Rotor angle thetam (rad),Electromagnetic torque Te (N*m)
  Measures : electricdrivelib/AC drives/PM Synchronous Motor Drive/Measures  SystemSampleTime=-1
  Mux : Subsystem
  SIm/SDL1 : driveline/Sensors & Actuators/Torque Actuator  SystemSampleTime=-1
  Speed Sensor : driveline/Sensors & Actuators/Motion Sensor  SystemSampleTime=-1  Angle=off  x0=0  Velocity=on  Acceleration=off
  Three-phase Inverter : powerlib/Power Electronics/Universal Bridge  SystemSampleTime=-1  Arms=3  SnubberResistance=5000  SnubberCapacitance=inf  Device=IGBT / Diodes  Ron=1e-3  Lon=0  ForwardVoltages="[  0  0  ]"  ForwardVoltage=0  GTOparameters=[ 10e-6 , 20e-6 ]  IGBTparameters=[ 1e-6 , 2e-6 ]*0  Measurements=None  Measurements_2=None  converterType=Rectifier
  Torque limitation : Subsystem
      mask Display: plot([0;1800;2000;2500;3000;3500], [1;1;0.90*1;0.72*1;0.6*1;0.51*1])
  VECT controller : Subsystem  mask(VECT){nb_p=4, dqInductances=[0.001597972349731   0.002057052250467], lambda=0.175666143629361, freq_max=20e3, Ts_vect=20e-6, h=0.1}
      mask prompts: nb_p "Motor pairs of poles"; dqInductances "Inductances [ Ld(H) Lq(H) ]:"; lambda "Flux induced by magnets (Wb)"; freq_max "Maximum switching frequency (Hz)"; Ts_vect "Sampling time (s)"; h "Current hysteresis bandwidth (A)"
      mask help: This block implements a vector controller.
      mask init: same as HEV_lib/Average-values/Motor Drive 50kW/VECT controller
      mask Display:
      | patch([X1 X1m],[Y1 Y1m],color1);
      | patch(X3,Y3,color2);
      | plot([X1 X1m X2 X2m X3 X4],[Y1 Y1m Y2 Y2m Y3 Y4]);
  +Vdc Bus : PMIOPort  Port=1  Side=Left
  -Vdc Bus : PMIOPort  Port=2  Side=Left
  Motor Shaft : PMIOPort  Port=3  Side=Right
  Motor : Outport
  Tem : Outport  Port=2
  wires:
  Ref Torque/1 -> Torque limitation/2(Torque)
  Torque limitation/1(torque) -> VECT controller/1(Torque*)
  Bus Selector/2 -> VECT controller/3(teta)  "<Rotor angle thetam (rad)>"
  Measures/1 -> VECT controller/4(I_abc)
  Bus Selector/1 -> Torque limitation/1(N rad/s), VECT controller/2(w)  "<Rotor speed wm (rad/s)>"
  Bus Selector/3 -> SIm/SDL1/1, Tem/1  "<Electromagnetic torque Te (N*m)>"
  500 Vdc 50kW PMSM/1 -> Motor/1, Bus Selector/1, Mux/2(m)
  Speed Sensor/1 -> 500 Vdc 50kW PMSM/1
  VECT controller/1(gates) -> Mux/1(gates)
  Mux/1(g) -> Three-phase Inverter/1
  connections:
  SIm/SDL1/RConn1 -- Motor Shaft/RConn1 -- Speed Sensor/LConn1
  -Vdc Bus/RConn1 -- Three-phase Inverter/RConn2
  +Vdc Bus/RConn1 -- Three-phase Inverter/RConn1
  Measures/RConn1 -- 500 Vdc 50kW PMSM/LConn1
  Measures/RConn2 -- 500 Vdc 50kW PMSM/LConn2
  Measures/RConn3 -- 500 Vdc 50kW PMSM/LConn3
  Three-phase Inverter/LConn1 -- Measures/LConn1
  Measures/LConn2 -- Three-phase Inverter/LConn2
  Three-phase Inverter/LConn3 -- Measures/LConn3

== system HEV_lib/Detailed/demux ==
  motor : Inport
  Ctrl : Inport  Port=2
  "+ -> -1" : Gain  Gain=30/pi
  Bus Selector : BusSelector  OutputSignals=Stator current is_a (A),Rotor speed wm (rad/s),Electromagnetic torque Te (N*m)
  Mux1 : Mux  Inputs=2
  i_a : Outport
  speed : Outport  Port=2
  Torque : Outport  Port=3
  wires:
  Bus Selector/1 -> i_a/1  "<Stator current is_a (A)>"
  Mux1/1 -> Torque/1
  Bus Selector/3 -> Mux1/1  "<Electromagnetic torque Te (N*m)>"
  Bus Selector/2 -> "+ -> -1"/1  "<Rotor speed wm (rad/s)>"
  Ctrl/1 -> Mux1/2
  motor/1 -> Bus Selector/1
  "+ -> -1"/1 -> speed/1

== system HEV_lib/Detailed/demux1 ==
  motor : Inport
  Ctrl : Inport  Port=2
  "+ -> -1" : Gain  Gain=30/pi
  Bus Selector : BusSelector  OutputSignals=Stator current is_a (A),Rotor speed wm (rad/s),Electromagnetic torque Te (N*m)
  Mux1 : Mux  Inputs=2
  i_a : Outport
  speed : Outport  Port=2
  Torque : Outport  Port=3
  wires:
  "+ -> -1"/1 -> speed/1
  motor/1 -> Bus Selector/1
  Bus Selector/1 -> i_a/1  "<Stator current is_a (A)>"
  Ctrl/1 -> Mux1/2
  Bus Selector/2 -> "+ -> -1"/1  "<Rotor speed wm (rad/s)>"
  Bus Selector/3 -> Mux1/1  "<Electromagnetic torque Te (N*m)>"
  Mux1/1 -> Torque/1

== system HEV_lib/Simplified/DC/DC Converter ==
  Break Alg Loop : TransferFcn  Denominator=[0.001 1]
  Constant : Constant  Value=500
  Controlled Current Source : powerlib/Electrical Sources/Controlled Current Source  SystemSampleTime=-1  Initialize=on  Source_Type=AC  Amplitude=0  Phase=0  Frequency=0  Measurements=None
  Controlled Voltage Source : powerlib/Electrical Sources/Controlled Voltage Source  SystemSampleTime=-1  Initialize=on  Source_Type=AC  Amplitude=0  Phase=0  Frequency=0  Measurements=None
  Current Measurement : powerlib/Measurements/Current Measurement  SystemSampleTime=-1  PhasorSimulation=off  OutputType=Complex  PSBequivalent=0
  Product : Product  Inputs=**/  RndMeth=Zero
  Voltage Measurement : powerlib/Measurements/Voltage Measurement  SystemSampleTime=-1  PhasorSimulation=off  OutputType=Complex  PSBequivalent=0
  Zero Avoider : Saturate  UpperLimit=inf  LowerLimit=1
  +Vdc Bus : PMIOPort  Tag=PMCPort  Port=1  Side=Right
  -Vdc Bus : PMIOPort  Tag=PMCPort  Port=2  Side=Right
  + battery : PMIOPort  Tag=PMCPort  Port=3  Side=Left
  - battery : PMIOPort  Tag=PMCPort  Port=4  Side=Left
  wires:
  Constant/1 -> Controlled Voltage Source/1, Product/2
  Product/1 -> Controlled Current Source/1
  Current Measurement/1 -> Product/1
  Voltage Measurement/1 -> Break Alg Loop/1
  Break Alg Loop/1 -> Zero Avoider/1
  Zero Avoider/1 -> Product/3
  connections:
  Current Measurement/LConn1 -- Controlled Voltage Source/RConn1
  Controlled Current Source/LConn1 -- + battery/RConn1 -- Voltage Measurement/LConn1
  - battery/RConn1 -- Controlled Current Source/RConn1 -- Voltage Measurement/LConn2
  Current Measurement/RConn1 -- +Vdc Bus/RConn1
  -Vdc Bus/RConn1 -- Controlled Voltage Source/LConn1

== system HEV_lib/Simplified/Electrical measurements ==
  Imot : Inport
  Vdc : Inport  Port=2
  m battery : Inport  Port=3
  Igen : Inport  Port=4
  Bus Selector : BusSelector  OutputSignals=Voltage (V),Current (A),SOC (%)
  Mux : Mux  Inputs=2
  Mux1 : Mux  Inputs=3
  Mux2 : Mux  Inputs=3
  Mux3 : Mux
  Mux4 : Mux  Inputs=2
  Product1 : Product  RndMeth=Zero
  Product2 : Product  RndMeth=Zero
  Product3 : Product  RndMeth=Zero
  tag scope: Electricals=global, Power=global
  wires:
  Product2/1 -> Mux1/1  "Motor Power (W)"
  Product1/1 -> Mux1/2  "Generator power (W)"
  Product3/1 -> Mux1/3  "Battery power (W)"
  Imot/1 -> Product2/1, Mux2/1
  Mux1/1 -> [Power]
  m battery/1 -> Bus Selector/1
  Bus Selector/1 -> Mux/2, Product3/1  "<Voltage (V)>"
  Bus Selector/2 -> Product3/2, Mux2/2  "<Current (A)>"
  Mux/1 -> Mux3/2  "Voltage (DC bus, Battery)"
  Mux2/1 -> Mux3/3  "Current (Motor, Battery, Generator)"
  Igen/1 -> Product1/1, Mux2/3
  Bus Selector/3 -> Mux3/4  "<SOC (%)>"
  Vdc/1 -> Product2/2, Product1/2, Mux/1, Mux4/1, Mux4/2
  Mux3/1 -> [Electricals]
  Mux4/1 -> Mux3/1

== system HEV_lib/Simplified/Generator Drive 30kW ==
  Ref Torque : Inport
  Break Alg Loop : TransferFcn  Denominator=[0.001 1]
  Controlled Current Source : powerlib/Electrical Sources/Controlled Current Source  SystemSampleTime=-1  Initialize=on  Source_Type=AC  Amplitude=0  Phase=0  Frequency=0  Measurements=None
  Product : Product  Inputs=**/  RndMeth=Zero
  SIm/SDL1 : driveline/Sensors & Actuators/Torque Actuator  SystemSampleTime=-1
  Speed Sensor : driveline/Sensors & Actuators/Motion Sensor  SystemSampleTime=-1  Angle=off  x0=0  Velocity=on  Acceleration=off
  Voltage Measurement : powerlib/Measurements/Voltage Measurement  SystemSampleTime=-1  PhasorSimulation=off  OutputType=Complex  PSBequivalent=0
  Zero Avoider : Saturate  UpperLimit=inf  LowerLimit=1
  +Vdc Bus : PMIOPort  Port=1  Side=Left
  -Vdc Bus : PMIOPort  Port=2  Side=Left
  Generator Shaft : PMIOPort  Port=3  Side=Right
  wires:
  Ref Torque/1 -> SIm/SDL1/1, Product/2
  Product/1 -> Controlled Current Source/1
  Voltage Measurement/1 -> Break Alg Loop/1
  Break Alg Loop/1 -> Zero Avoider/1
  Zero Avoider/1 -> Product/3
  Speed Sensor/1 -> Product/1
  connections:
  Voltage Measurement/LConn1 -- +Vdc Bus/RConn1 -- Controlled Current Source/LConn1
  Voltage Measurement/LConn2 -- Controlled Current Source/RConn1 -- -Vdc Bus/RConn1
  Speed Sensor/LConn1 -- SIm/SDL1/RConn1 -- Generator Shaft/RConn1

== system HEV_lib/Simplified/Meas VI3 ==
  V1 : powerlib/Measurements/Voltage Measurement  SystemSampleTime=-1  PhasorSimulation=off  OutputType=Complex  PSBequivalent=0
  i1 : powerlib/Measurements/Current Measurement  SystemSampleTime=-1  PhasorSimulation=off  OutputType=Complex  PSBequivalent=0
  iref : PMIOPort  Port=1  Side=Right
  + : PMIOPort  Tag=PMCPort  Port=2  Side=Left
  vref : PMIOPort  Port=3  Side=Left
  iout : Outport
  vout : Outport  Port=2
  wires:
  V1/1 -> vout/1
  i1/1 -> iout/1
  connections:
  vref/RConn1 -- V1/LConn2
  iref/RConn1 -- i1/RConn1
  i1/LConn1 -- +/RConn1 -- V1/LConn1

== system HEV_lib/Simplified/Motor Drive 50kW ==
  Ref Torque : Inport
  Break Alg Loop : TransferFcn  Denominator=[0.001 1]
  Controlled Current Source : powerlib/Electrical Sources/Controlled Current Source  SystemSampleTime=-1  Initialize=on  Source_Type=AC  Amplitude=0  Phase=0  Frequency=0  Measurements=None
  Product : Product  Inputs=**/  RndMeth=Zero
  SIm/SDL1 : driveline/Sensors & Actuators/Torque Actuator  SystemSampleTime=-1
  Speed Sensor : driveline/Sensors & Actuators/Motion Sensor  SystemSampleTime=-1  Angle=off  x0=0  Velocity=on  Acceleration=off
  Voltage Measurement : powerlib/Measurements/Voltage Measurement  SystemSampleTime=-1  PhasorSimulation=off  OutputType=Complex  PSBequivalent=0
  Zero Avoider : Saturate  UpperLimit=inf  LowerLimit=1
  +Vdc Bus : PMIOPort  Port=1  Side=Left
  -Vdc Bus : PMIOPort  Port=2  Side=Left
  Motor Shaft : PMIOPort  Port=3  Side=Right
  wires:
  Ref Torque/1 -> SIm/SDL1/1, Product/2
  Product/1 -> Controlled Current Source/1
  Voltage Measurement/1 -> Break Alg Loop/1
  Break Alg Loop/1 -> Zero Avoider/1
  Zero Avoider/1 -> Product/3
  Speed Sensor/1 -> Product/1
  connections:
  +Vdc Bus/RConn1 -- Controlled Current Source/LConn1 -- Voltage Measurement/LConn1
  Controlled Current Source/RConn1 -- -Vdc Bus/RConn1 -- Voltage Measurement/LConn2
  SIm/SDL1/RConn1 -- Motor Shaft/RConn1 -- Speed Sensor/LConn1

== system HEV_lib/Average-values/DC/DC Converter/Average-values Boost Converter ==
  Duty Cycle : Inport
  Average-value armature voltage : Fcn  Expr=u(1)*u(2)
  Average-value source current : Fcn  Expr=u(1)*u(2)
  Controlled Current Source : powerlib/Electrical Sources/Controlled Current Source  SystemSampleTime=-1  Initialize=on  Source_Type=AC  Amplitude=0  Phase=0  Frequency=0  Measurements=None
  Controlled Voltage Source : powerlib/Electrical Sources/Controlled Voltage Source  SystemSampleTime=-1  Initialize=on  Source_Type=AC  Amplitude=0  Phase=0  Frequency=0  Measurements=None
  Current Measurement : powerlib/Measurements/Current Measurement  Tag=PoWeRsYsTeMmEaSuReMeNt  SystemSampleTime=-1  PhasorSimulation=off  OutputType=Magnitude  PSBequivalent=0
  Mux : Mux  Inputs=2
  Mux1 : Mux  Inputs=2
  Selector : Selector  InputPortWidth=2  IndexOptions=Index vector (dialog)  Indices=[1]  OutputSizes=1
  Unit Delay : UnitDelay  SampleTime=Ts
  Unit Delay1 : UnitDelay  SampleTime=Ts
  Voltage Measurement1 : powerlib/Measurements/Voltage Measurement  Tag=PoWeRsYsTeMmEaSuReMeNt  SystemSampleTime=-1  PhasorSimulation=off  OutputType=Magnitude  PSBequivalent=0
  A : PMIOPort  Port=1  Side=Right
  + : PMIOPort  Port=2  Side=Left
  - : PMIOPort  Port=3  Side=Left
  wires:
  Selector/1 -> Mux1/1, Mux/1
  Unit Delay1/1 -> Controlled Current Source/1
  Average-value source current/1 -> Unit Delay1/1
  Current Measurement/1 -> Mux1/2
  Mux1/1 -> Average-value source current/1
  Duty Cycle/1 -> Selector/1
  Voltage Measurement1/1 -> Mux/2
  Mux/1 -> Average-value armature voltage/1
  Average-value armature voltage/1 -> Unit Delay/1
  Unit Delay/1 -> Controlled Voltage Source/1
  connections:
  A/RConn1 -- Current Measurement/RConn1
  Controlled Voltage Source/RConn1 -- Current Measurement/LConn1
  +/RConn1 -- Voltage Measurement1/LConn1 -- Controlled Current Source/LConn1
  Controlled Voltage Source/LConn1 -- -/RConn1 -- Controlled Current Source/RConn1 -- Voltage Measurement1/LConn2

== system HEV_lib/Average-values/DC/DC Converter/Current controller DISCRETE3 ==
  Uref : Inport
  UBus : Inport  Port=2
  Clock1 : Clock
      settings: Decimation=10
  Compare To Constant1 : simulink/Logic and Bit Operations/Compare To Constant  SystemSampleTime=-1  relop=>  const=0.01  LogicOutDataTypeMode=uint8  ZeroCross=off
  Ctrl sat. : Saturate  UpperLimit=0.95  LowerLimit=-0.95
  Discrete-Time Integrator : DiscreteIntegrator  IntegratorMethod=Integration: Trapezoidal  SampleTime=Ts  LimitOutput=on  UpperSaturationLimit=1  LowerSaturationLimit=-1  ICPrevOutput=DiscIntNeverNeededParam  ICPrevScaledInput=DiscIntNeverNeededParam
  Integral gain : Gain  Gain=Ki  SaturateOnIntegerOverflow=on  OutDataTypeStr=Inherit: Same as input  ParamDataTypeStr=Inherit: Same as input
  Product1 : Product  RndMeth=Zero
  Proportional gain : Gain  Gain=Kp  SaturateOnIntegerOverflow=on  OutDataTypeStr=Inherit: Same as input  ParamDataTypeStr=Inherit: Same as input
  Sum1 : Sum  Inputs=+-  SaturateOnIntegerOverflow=on  InputSameDT=on  OutDataTypeStr=Inherit: Same as first input
  Sum2 : Sum  SaturateOnIntegerOverflow=on  InputSameDT=on  OutDataTypeStr=Inherit: Same as first input
  Transfer Fcn : TransferFcn  Denominator=[.0001 1]
  Zero-Order Hold1 : ZeroOrderHold  SampleTime=Ts
  Ec : Outport  InitialOutput=0
  wires:
  Uref/1 -> Sum1/2
  Transfer Fcn/1 -> Sum1/1
  Zero-Order Hold1/1 -> Transfer Fcn/1
  Product1/1 -> Proportional gain/1, Integral gain/1
  Compare To Constant1/1 -> Product1/2
  Clock1/1 -> Compare To Constant1/1
  Sum1/1 -> Product1/1
  Ctrl sat./1 -> Ec/1
  Proportional gain/1 -> Sum2/1
  Integral gain/1 -> Discrete-Time Integrator/1
  UBus/1 -> Zero-Order Hold1/1
  Discrete-Time Integrator/1 -> Sum2/2
  Sum2/1 -> Ctrl sat./1

== system HEV_lib/Average-values/DC/DC Converter/Duty Cycles ==
  Ec : Inport
  Add : Sum  Inputs=+-
  Bus Creator2 : BusCreator  Inputs=2
  Constant : Constant
  Duty Cycle : Fcn  Expr=0.5*(u[1]+1)
  Unit Delay2 : UnitDelay  X0=.5  SampleTime=Ts
  dc : Outport
  wires:
  Unit Delay2/1 -> dc/1
  Duty Cycle/1 -> Add/2, Bus Creator2/1  "IGBT I"
  Add/1 -> Bus Creator2/2  "IGBT 2"
  Constant/1 -> Add/1
  Ec/1 -> Duty Cycle/1
  Bus Creator2/1 -> Unit Delay2/1

== system HEV_lib/Average-values/Generator Drive 30kW/Mux ==
  sig* : Inport
  m : Inport  Port=2
  Bus Creator : BusCreator  Inputs=2
  Ctrl : Outport
  wires:
  m/1 -> Bus Creator/2  "m"
  sig*/1 -> Bus Creator/1  "Signals*"
  Bus Creator/1 -> Ctrl/1
